simulink model "sampleModel142new"  (R2021b)
settings: Solver=VariableStepAuto  StartTime=0.0  StopTime=10.0  RelTol=1e-3
undefined symbols (not defined in the file): magnitude, Newton, Raphson
libraries: simulink x9
settings Model: Creator=user  LastModifiedBy=cemery

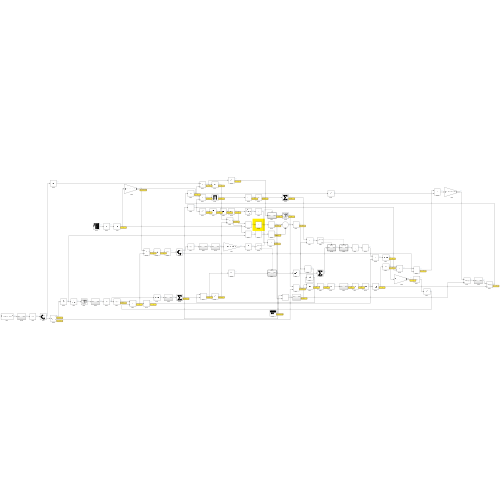
[thumbnail: Simulink's stored preview of the top-level diagram]
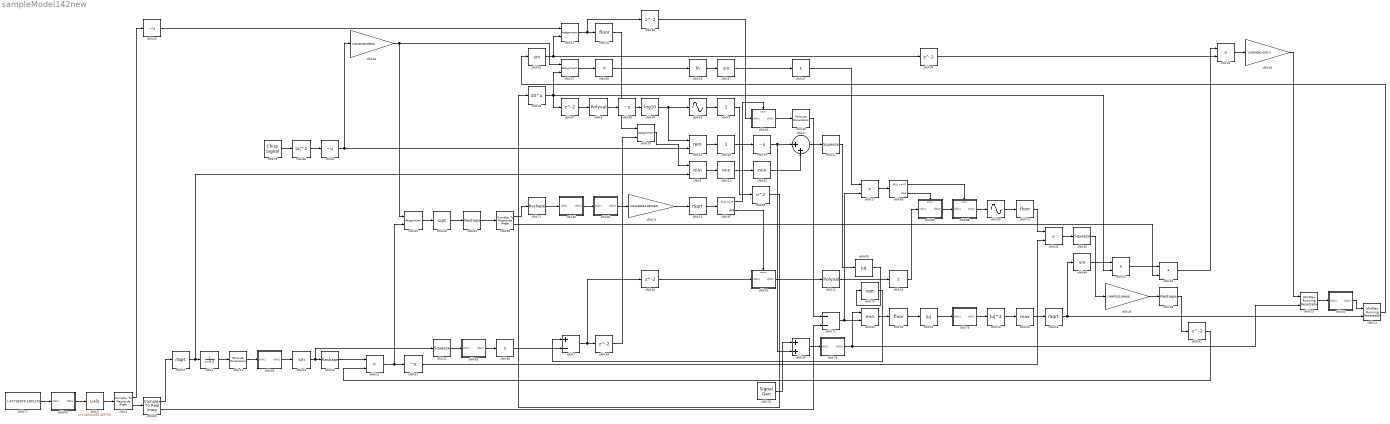
== system sampleModel142new ==
  cfblk1 : DiscreteTransferFcn  SampleTime=1
  cfblk10 : Rounding
  cfblk11 : simulink/Math Operations/MinMax Running Resettable  Function=min  vinit=0.0
  cfblk12 : Polyval  Coefs=[ +2.081618890e-019, -1.441693666e-014, +4.719686976e-010, -8.536869453e-006, +1.621573104e-001, -8.087801117e+001 ]
  cfblk13 : Math  Operator=magnitude^2  SaturateOnIntegerOverflow=on
  cfblk14 : Sum  Inputs=+
  cfblk15 : Sqrt  Operator=rSqrt  AlgorithmType=Newton-Raphson  SaturateOnIntegerOverflow=on
  cfblk16 : Sqrt  Operator=rSqrt  AlgorithmType=Newton-Raphson  SaturateOnIntegerOverflow=on
  cfblk{17,24,43,50} (4 alike) : Product  Inputs=**
  cfblk{18,22,67,71} (4 alike) : Reshape
  cfblk19 : MinMax  Function=max
  cfblk2 : Sum  Inputs=|++
  cfblk20 : Math  Operator=10^u  SaturateOnIntegerOverflow=on
  cfblk21 : MinMax
  cfblk23 : simulink/Math Operations/MinMax Running Resettable  Function=min  vinit=0.0
  cfblk{8,25,39,61,98} (5 alike) : UnaryMinus
  cfblk26 : Sqrt  SaturateOnIntegerOverflow=on
  cfblk{27,30,35,63} (4 alike) : Assignment  DiagnosticForDimensions=Warning  IndexOptions=Index vector (dialog)  Indices=1  OutputSizes=1
  cfblk28 : Gain  Gain=[243304992.433317]
  cfblk29 : Math  Operator=log  SaturateOnIntegerOverflow=on
  cfblk3 : Bias  Bias=[-438342693.429770]
  cfblk31 : Product
  cfblk32 : Squeeze
  cfblk33 : DotProduct  InputSameDT=on  OutDataTypeStr=Inherit: Inherit via internal rule
  cfblk36 : Sum
  cfblk{37,44,46,52} (4 alike) : Trigonometry
  cfblk38 : PermuteDimensions
  cfblk4 : ComplexToMagnitudeAngle
  cfblk40 : Squeeze
  cfblk41 : PermuteDimensions
  cfblk42 : Squeeze
  cfblk45 : Gain  Gain=[348875315.364563]
  cfblk47 : Sum  Inputs=+
  cfblk48 : simulink/Math Operations/Slider Gain  gain=1  low=0  high=2
  cfblk49 : Math  Operator=log10  SaturateOnIntegerOverflow=on
  cfblk5 : MinMax  Inputs=2
  cfblk51 : Abs
  cfblk53 : MinMax  Inputs=2
  cfblk54 : Rounding
  cfblk55 : Sin  TimeSource=Use external signal  SampleTime=0
  cfblk56 : Sin  TimeSource=Use external signal  SampleTime=0
  cfblk57 : Sqrt  Operator=rSqrt  AlgorithmType=Newton-Raphson  SaturateOnIntegerOverflow=on
  cfblk58 : ComplexToMagnitudeAngle
  cfblk59 : Math  Operator=square  SaturateOnIntegerOverflow=on
  cfblk6 : Polyval  Coefs=[ +2.081618890e-019, -1.441693666e-014, +4.719686976e-010, -8.536869453e-006, +1.621573104e-001, -8.087801117e+001 ]
  cfblk60 : Product  Inputs=*
  cfblk62 : MinMax
  cfblk64 : Gain  Gain=[202163136.326601]
  cfblk65 : Math  Operator=rem  SaturateOnIntegerOverflow=on
  cfblk66 : Math  Operator=magnitude^2  SaturateOnIntegerOverflow=on
  cfblk68 : Sum  Inputs=+
  cfblk69 : ComplexToRealImag
  cfblk7 : Sum  Inputs=+-
  cfblk70 : Sqrt  SaturateOnIntegerOverflow=on
  cfblk72 : Sum  Inputs=--
  cfblk73 : Rounding
  cfblk74 : Gain  Gain=[324436033.865340]
  cfblk75 : simulink/Sources/Chirp Signal  f1=[566895057.226011]  T=[-578514329.112329]  f2=[555426726.387373]
  cfblk76 : SignalGenerator  Amplitude=[511915908.876749]
  cfblk77 : Constant  Value=[-47735079.180120]  SampleTime=1
  cfblk78 : Subsystem
  cfblk79 : Subsystem
  cfblk80 : Subsystem
  cfblk81 : Subsystem
  cfblk82 : Subsystem
  cfblk83 : Subsystem
  cfblk84 : Subsystem
  cfblk85 : Subsystem
  cfblk86 : If  IfExpression=u1 >= 0  SampleTime=1
  cfblk87 : If  IfExpression=u1 >= 0  SampleTime=1
  cfblk88 : Subsystem  TreatAsAtomicUnit=on
  cfblk89 : Subsystem  TreatAsAtomicUnit=on
  cfblk9 : simulink/Math Operations/Slider Gain  gain=1  low=0  high=2
  cfblk90 : Subsystem  TreatAsAtomicUnit=on
  cfblk91 : Subsystem  TreatAsAtomicUnit=on
  cfblk{92..97} (6 alike) : Delay  SampleTime=1
  cfblk99 : Abs
  wires:
  cfblk72/1 -> cfblk17/2, cfblk53/2
  cfblk97/1 -> cfblk6/1
  cfblk92/1 -> cfblk31/2
  cfblk96/1 -> cfblk24/2
  cfblk21/1 -> cfblk62/1
  cfblk56/1 -> cfblk73/1
  cfblk93/1 -> cfblk90/1(cfblk1)
  cfblk79/1(cfblk2) -> cfblk13/1
  cfblk95/1 -> cfblk91/1(cfblk1)
  cfblk94/1 -> cfblk30/2
  cfblk13/1 -> cfblk19/1
  cfblk18/1 -> cfblk92/1
  cfblk15/1 -> cfblk87/1
  cfblk75/1 -> cfblk66/1
  cfblk87/2 -> cfblk91/Action
  cfblk55/1 -> cfblk9/1
  cfblk87/1 -> cfblk90/Action
  cfblk86/2 -> cfblk89/Action
  cfblk86/1 -> cfblk88/Action
  cfblk89/1(cfblk2) -> cfblk88/1(cfblk1)
  cfblk60/1 -> cfblk29/1
  cfblk25/1 -> cfblk63/1
  cfblk69/2 -> cfblk72/2
  cfblk36/1 -> cfblk78/1(cfblk1)
  cfblk71/1 -> cfblk82/1(cfblk1)
  cfblk53/1 -> cfblk54/1
  cfblk5/1 -> cfblk21/1
  cfblk47/1 -> cfblk17/1
  cfblk68/1 -> cfblk7/2
  cfblk45/1 -> cfblk18/1
  cfblk69/1 -> cfblk57/1
  cfblk37/1 -> cfblk47/1
  cfblk80/1(cfblk2) -> cfblk3/1
  cfblk58/2 -> cfblk33/2
  cfblk10/1 -> cfblk30/1
  cfblk62/1 -> cfblk2/2
  cfblk40/1 -> cfblk45/1
  cfblk9/1 -> cfblk59/1
  cfblk41/1 -> cfblk85/1(cfblk1)
  cfblk76/1 -> cfblk36/1
  cfblk38/1 -> cfblk72/1
  cfblk4/2 -> cfblk69/1
  cfblk3/1 -> cfblk4/1
  cfblk43/1 -> cfblk40/1
  cfblk51/1 -> cfblk79/1(cfblk1)
  cfblk33/1 -> cfblk24/1
  cfblk14/1 -> cfblk89/1(cfblk1)
  cfblk84/1(cfblk2) -> cfblk11/1
  cfblk83/1(cfblk2) -> cfblk68/1
  cfblk1/1 -> cfblk41/1
  cfblk73/1 -> cfblk43/1
  cfblk70/1 -> cfblk7/1
  cfblk65/1 -> cfblk48/1
  cfblk30/1 -> cfblk5/1
  cfblk61/1 -> cfblk43/2
  cfblk20/1 -> cfblk27/2, cfblk97/1, cfblk50/2
  cfblk82/1(cfblk2) -> cfblk81/1(cfblk1)
  cfblk27/1 -> cfblk60/1
  cfblk11/1 -> cfblk52/1
  cfblk2/1 -> cfblk42/1
  cfblk67/1 -> cfblk58/1
  cfblk24/1 -> cfblk28/1
  cfblk28/1 -> cfblk23/1
  cfblk90/1(cfblk2) -> cfblk38/1
  cfblk12/1 -> cfblk14/1
  cfblk50/1 -> cfblk33/1
  cfblk66/1 -> cfblk8/1
  cfblk46/1 -> cfblk50/1
  cfblk74/1 -> cfblk15/1
  cfblk85/1(cfblk2) -> cfblk44/1
  cfblk6/1 -> cfblk98/1
  cfblk23/1 -> cfblk84/1(cfblk1)
  cfblk26/1 -> cfblk67/1
  cfblk35/1 -> cfblk26/1
  cfblk29/1 -> cfblk37/1
  cfblk81/1(cfblk2) -> cfblk74/1
  cfblk22/1 -> cfblk31/1
  cfblk48/1 -> cfblk39/1
  cfblk54/1 -> cfblk51/1
  cfblk58/1 -> cfblk71/1
  cfblk91/1(cfblk2) -> cfblk12/1
  cfblk19/1 -> cfblk16/1
  cfblk59/1 -> cfblk20/1
  cfblk42/1 -> cfblk99/1
  cfblk77/1 -> cfblk80/1(cfblk1)
  cfblk88/1(cfblk2) -> cfblk56/1
  cfblk32/1 -> cfblk83/1(cfblk1)
  cfblk4/1 -> cfblk25/1
  cfblk17/1 -> cfblk86/1
  cfblk64/1 -> cfblk35/1, cfblk27/1
  cfblk52/1 -> cfblk63/2, cfblk96/1
  cfblk7/1 -> cfblk94/1, cfblk95/1
  cfblk8/1 -> cfblk64/1, cfblk65/2
  cfblk63/1 -> cfblk10/1, cfblk93/1
  cfblk57/1 -> cfblk1/1, cfblk5/2
  cfblk31/1 -> cfblk61/1, cfblk35/2
  cfblk49/1 -> cfblk55/1, cfblk65/1
  cfblk78/1(cfblk2) -> cfblk53/1, cfblk23/2
  cfblk16/1 -> cfblk46/1, cfblk11/2
  cfblk39/1 -> cfblk2/1, cfblk36/2
  cfblk44/1 -> cfblk22/1, cfblk32/1
  cfblk98/1 -> cfblk49/1
  cfblk99/1 -> cfblk70/1

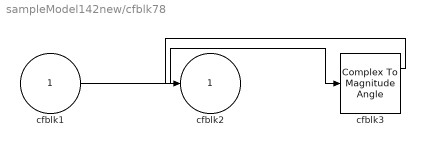
== system sampleModel142new/cfblk78 ==
  cfblk1 : Inport
  cfblk3 : ComplexToMagnitudeAngle
  cfblk2 : Outport
  wires:
  cfblk1/1 -> cfblk3/1
  cfblk3/1 -> cfblk2/1

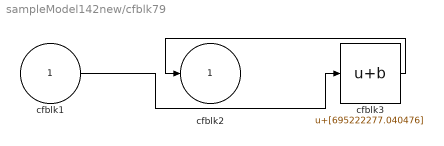
== system sampleModel142new/cfblk79 ==
  cfblk1 : Inport
  cfblk3 : Bias  Bias=[695222277.040476]
  cfblk2 : Outport
  wires:
  cfblk3/1 -> cfblk2/1
  cfblk1/1 -> cfblk3/1

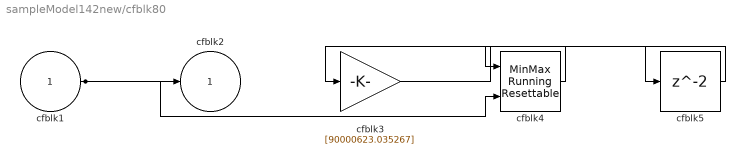
== system sampleModel142new/cfblk80 ==
  cfblk1 : Inport
  cfblk3 : Gain  Gain=[90000623.035267]
  cfblk4 : simulink/Math Operations/MinMax Running Resettable  Function=min  vinit=0.0
  cfblk5 : Delay  SampleTime=1
  cfblk2 : Outport
  wires:
  cfblk1/1 -> cfblk2/1, cfblk4/2
  cfblk4/1 -> cfblk3/1
  cfblk3/1 -> cfblk5/1
  cfblk5/1 -> cfblk4/1

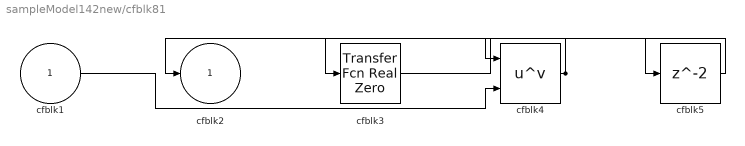
== system sampleModel142new/cfblk81 ==
  cfblk1 : Inport
  cfblk3 : simulink/Discrete/Transfer Fcn Real Zero  ZeroZ=0.75  ICPrevInput=0.0  DoSatur=off
      settings: SourceProductBaseCode=SL
  cfblk4 : Math  Operator=pow  SaturateOnIntegerOverflow=on
  cfblk5 : Delay  SampleTime=1
  cfblk2 : Outport
  wires:
  cfblk4/1 -> cfblk2/1, cfblk3/1
  cfblk1/1 -> cfblk4/2
  cfblk3/1 -> cfblk5/1
  cfblk5/1 -> cfblk4/1

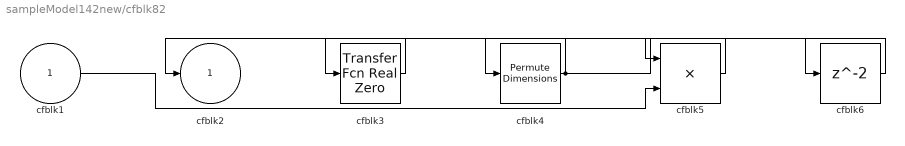
== system sampleModel142new/cfblk82 ==
  cfblk1 : Inport
  cfblk3 : simulink/Discrete/Transfer Fcn Real Zero  ZeroZ=0.75  ICPrevInput=0.0  DoSatur=off
      settings: SourceProductBaseCode=SL
  cfblk4 : PermuteDimensions
  cfblk5 : Product
  cfblk6 : Delay  SampleTime=1
  cfblk2 : Outport
  wires:
  cfblk4/1 -> cfblk3/1, cfblk6/1
  cfblk3/1 -> cfblk2/1
  cfblk1/1 -> cfblk5/2
  cfblk5/1 -> cfblk4/1
  cfblk6/1 -> cfblk5/1

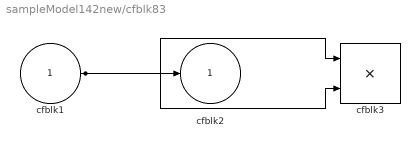
== system sampleModel142new/cfblk83 ==
  cfblk1 : Inport
  cfblk3 : Product  Inputs=**
  cfblk2 : Outport
  wires:
  cfblk1/1 -> cfblk2/1, cfblk3/1, cfblk3/2

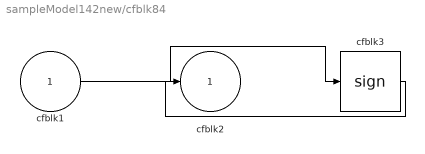
== system sampleModel142new/cfblk84 ==
  cfblk1 : Inport
  cfblk3 : Signum
  cfblk2 : Outport
  wires:
  cfblk1/1 -> cfblk3/1
  cfblk3/1 -> cfblk2/1

== system sampleModel142new/cfblk85 ==
  cfblk1 : Inport
  cfblk3 : Abs
  cfblk2 : Outport
  wires:
  cfblk1/1 -> cfblk3/1
  cfblk3/1 -> cfblk2/1

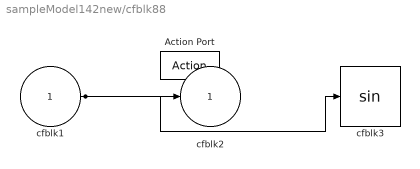
== system sampleModel142new/cfblk88 ==
  cfblk1 : Inport
  Action Port : ActionPort  ActionPortLabel=if(u1 >= 0)
  cfblk3 : Trigonometry
  cfblk2 : Outport
  wires:
  cfblk1/1 -> cfblk2/1, cfblk3/1

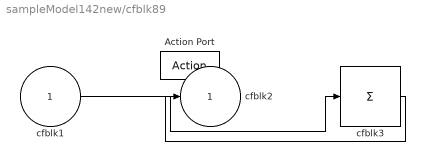
== system sampleModel142new/cfblk89 ==
  cfblk1 : Inport
  Action Port : ActionPort  ActionPortLabel=else
  cfblk3 : Sum  Inputs=+
  cfblk2 : Outport
  wires:
  cfblk1/1 -> cfblk3/1
  cfblk3/1 -> cfblk2/1

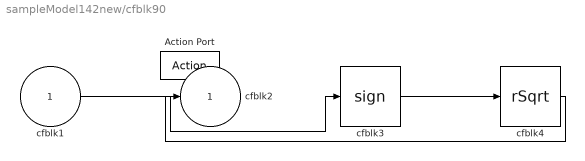
== system sampleModel142new/cfblk90 ==
  cfblk1 : Inport
  Action Port : ActionPort  ActionPortLabel=if(u1 >= 0)
  cfblk3 : Signum
  cfblk4 : Sqrt  Operator=rSqrt  AlgorithmType=Newton-Raphson  SaturateOnIntegerOverflow=on
  cfblk2 : Outport
  wires:
  cfblk1/1 -> cfblk3/1
  cfblk3/1 -> cfblk4/1
  cfblk4/1 -> cfblk2/1

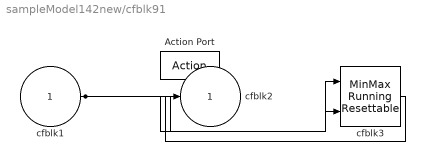
== system sampleModel142new/cfblk91 ==
  cfblk1 : Inport
  Action Port : ActionPort  ActionPortLabel=else
  cfblk3 : simulink/Math Operations/MinMax Running Resettable  Function=min  vinit=0.0
  cfblk2 : Outport
  wires:
  cfblk1/1 -> cfblk3/1, cfblk3/2
  cfblk3/1 -> cfblk2/1
